simulink model "acc"  (R2015a)
settings: Solver=ode113  StartTime=0.0  StopTime=20  FixedStep=.00001  RelTol=1e-9
undefined symbols (not defined in the file or in its folder): Grx, rrx
libraries: cstblocks x6, simulink x1
settings Model: Creator=morten  LastModifiedBy=roevhat
settings SolverCC: SolverJacobianMethodControl=FullPerturbation  AlgebraicLoopSolver=LineSearch
settings ModelReferenceCC: ModelReferenceMinAlgLoopOccurrences=on

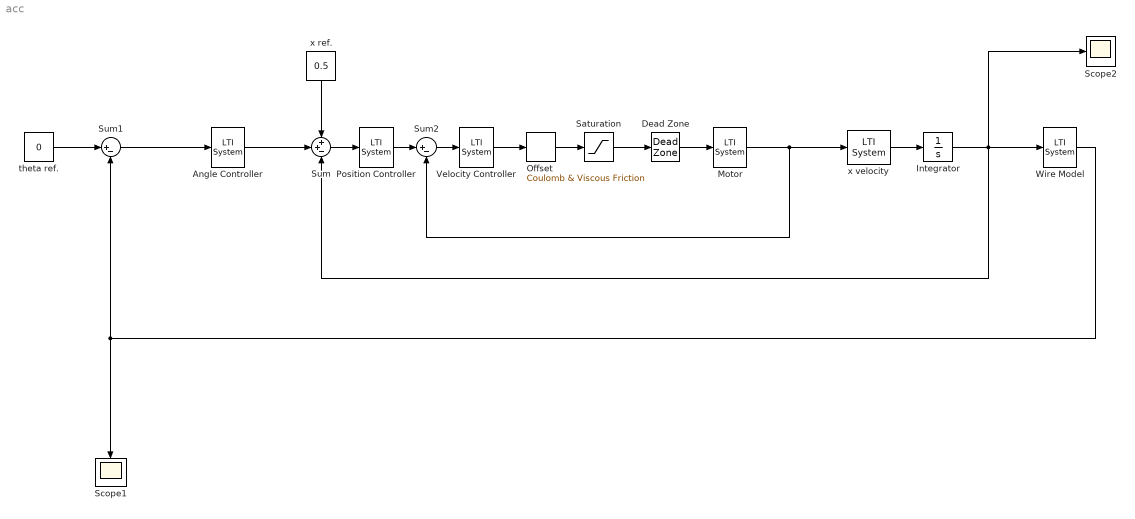
== system acc ==
  Angle Controller : cstblocks/LTI System  sys=C2  IC=[]
  Dead Zone : DeadZone  LowerValue=-4.5  UpperValue=4.5  SaturateOnIntegerOverflow=on
  Integrator : Integrator
  Motor : cstblocks/LTI System  sys=Mx  IC=[]
  Offset : simulink/Discontinuities/Coulomb & Viscous Friction  offset=4.5  gain=1
  Position Controller : cstblocks/LTI System  sys=C1  IC=[]
  Saturation : Saturate  UpperLimit=12.5  LowerLimit=-12.5
  Scope1 : Scope
      settings: TimeRange=20  YMin=-0.03  YMax=0.03
  Scope2 : Scope
      settings: TimeRange=20  YMin=-0.03  YMax=0.03
  Sum : Sum  Inputs=++-
  Sum1 : Sum  Inputs=|+-
  Sum2 : Sum  Inputs=|+-
  Velocity Controller : cstblocks/LTI System  sys=C0  IC=[]
  Wire Model : cstblocks/LTI System  sys=W  IC=[]
  theta ref. : Constant  Value=0
  x ref. : Constant  Value=0.5
  x velocity : cstblocks/LTI System  sys=Grx * rrx  IC=[]
  wires:
  theta ref./1 -> Sum1/1
  Offset/1 -> Saturation/1
  Sum1/1 -> Angle Controller/1
  Wire Model/1 -> Sum1/2, Scope1/1
  Sum/1 -> Position Controller/1
  Dead Zone/1 -> Motor/1
  Angle Controller/1 -> Sum/2
  x velocity/1 -> Integrator/1
  Saturation/1 -> Dead Zone/1
  x ref./1 -> Sum/1
  Motor/1 -> Sum2/2, x velocity/1
  Integrator/1 -> Scope2/1, Wire Model/1, Sum/3
  Position Controller/1 -> Sum2/1
  Sum2/1 -> Velocity Controller/1
  Velocity Controller/1 -> Offset/1
